simulink model "TSR_Scenario_001_cs"  (R2014b)
settings: Solver=ode5  SolverMode=SingleTasking  StartTime=0.0  StopTime=inf  FixedStep=1/100  RelTol=1e-3
PreLoadFcn:
  | mbxruntime.callbacks.PreLoadFcn(bdroot);
  | check_NUTS_defined;
  | 
  | assignin('base',['model_closed_' bdroot],false);
  | 
  | addpath('../includes_TSR/includes_TSR');
  | 
  | switch version('-release')
  | case {'2010a', '2010b', '2011a'}
  | addpath('../includes_TSR/ML2010b');
  | otherwise
  | addpath('../includes_TSR/ML2011b');
  | end
PostLoadFcn:
  | mbxruntime.callbacks.PostLoadFcn(bdroot);
InitFcn:
  | mbxruntime.callbacks.InitFcn(bdroot);
StartFcn:
  | mbxruntime.callbacks.StartFcn(bdroot);
StopFcn:
  | mbxruntime.callbacks.StopFcn(bdroot);
model workspace: external: MAT-File .\TSR_Scenario_001_cs_hws.mat (data not in the file)
undefined symbols (not defined in the file or in its folder): InitImageOutputDir, mbxruntime, OrientationPitch, OrientationRoll, PositionX, PositionY, PositionZ, tabledata, warningInitialVelocity, x0
undefined symbols (not defined in the file): SteeringColumn, SteeringWheel, TSR_Scenario_001_cs_0469e6db089af631, TSR_Scenario_001_cs_0511100212e7bc8e, TSR_Scenario_001_cs_0e7e9ae969427aac, TSR_Scenario_001_cs_1093386e49c2fe1f, TSR_Scenario_001_cs_112063adae8cf595, TSR_Scenario_001_cs_20f00d93cd5331c2, TSR_Scenario_001_cs_23e3512474fbfadc, TSR_Scenario_001_cs_366523e1554c6bf4, TSR_Scenario_001_cs_37bce4982c67337a, TSR_Scenario_001_cs_44e6164a5df50f45, TSR_Scenario_001_cs_4963ce12e7ff3247, TSR_Scenario_001_cs_4b3e01fa729ce73a, TSR_Scenario_001_cs_519c34727ce9f069, TSR_Scenario_001_cs_5b66ab60038399a1, TSR_Scenario_001_cs_5baa165dfa1afdcb, TSR_Scenario_001_cs_5f993ce39fa6372c, TSR_Scenario_001_cs_613fdf28e3ff7437, TSR_Scenario_001_cs_67b1406af835d622, TSR_Scenario_001_cs_6ad990c290286b94, TSR_Scenario_001_cs_6c412b69295984e1, TSR_Scenario_001_cs_6d4c0c06b1585ef3, TSR_Scenario_001_cs_6dd019d071bf1235, TSR_Scenario_001_cs_6e9f5883f1a78533, TSR_Scenario_001_cs_80f7223d9ac35404, TSR_Scenario_001_cs_8562b82d3c89ae57, TSR_Scenario_001_cs_8a3a0181ab0babfe, TSR_Scenario_001_cs_8c997348ce80deaf, TSR_Scenario_001_cs_925bd6a073d9fe25, TSR_Scenario_001_cs_961436216add6114, TSR_Scenario_001_cs_991a7959256b2c84, TSR_Scenario_001_cs_9a95ce2c2e753616, TSR_Scenario_001_cs_a98aa9562e8552a9, TSR_Scenario_001_cs_ab44ae81dbfb58cd, TSR_Scenario_001_cs_Actros_2541_2_Path_pathUniqueID, TSR_Scenario_001_cs_ae74836ade6bff5a, TSR_Scenario_001_cs_Audi_A8_1_Dynamics_Simple_initialPitch, TSR_Scenario_001_cs_Audi_A8_1_Dynamics_Simple_initialRoll, TSR_Scenario_001_cs_Audi_A8_1_Dynamics_Simple_initialX, TSR_Scenario_001_cs_Audi_A8_1_Dynamics_Simple_initialY, TSR_Scenario_001_cs_Audi_A8_1_Dynamics_Simple_initialYaw, TSR_Scenario_001_cs_Audi_A8_1_Dynamics_Simple_initialZ, TSR_Scenario_001_cs_Audi_A8_2_Path_pathUniqueID, TSR_Scenario_001_cs_Audi_A8_2_SpeedProfile_speedProfileUniqueID, TSR_Scenario_001_cs_b2eca4eb2fce349a, TSR_Scenario_001_cs_b7bac209c1f2549f, TSR_Scenario_001_cs_bf3dccb66d3255a4, TSR_Scenario_001_cs_bf4c1a5315e3f716, TSR_Scenario_001_cs_BMW_Z3_1_Path_pathUniqueID, TSR_Scenario_001_cs_BMW_Z3_1_SpeedProfile_speedProfileUniqueID, TSR_Scenario_001_cs_BMW_Z3_2_Path_pathUniqueID, TSR_Scenario_001_cs_BMW_Z3_2_SpeedProfile_speedProfileUniqueID, TSR_Scenario_001_cs_c4c8fc4bdece03a9, TSR_Scenario_001_cs_c964c86aa54ad92e, TSR_Scenario_001_cs_cb64d1ef85329755, TSR_Scenario_001_cs_Citroen_C3_1_Path_pathUniqueID, TSR_Scenario_001_cs_Citroen_C3_2_Path_pathUniqueID, TSR_Scenario_001_cs_Citroen_C3_3_Path_pathUniqueID, TSR_Scenario_001_cs_Citroen_C3_4_Path_pathUniqueID ... (+25)
libraries: simulink x21, PreScanSimulinkLibrary x17, simulink_extras x13
(part 14 of 30)

== system TSR_Scenario_001_cs/VISUMatrixSignLights_HighwayOverhang_2/Actuator ==
  VISUMatrixSignLights_HighwayOverhang_2 : Inport  Tag=inport/VisuMatrixSignLights  SampleTime=1/100  BusOutputAsStruct=on
  DemuxVisuLights : Demux  Outputs=16
  LimiterVisuLights : Saturate  UpperLimit=1  LowerLimit=0
  visu_MatrixSign_5_Light_1 : S-Function  FunctionName=sfun_MaterialColorSelector  Parameters=mbxruntime.parameters.convert(UniqueID), mbxruntime.parameters.convert(ColorsObjectQuery), mbxruntime.parameters.convert(Colors),tabledata, TimeStep  EnableBusSupport=off  mask(PreScan Sink Block: VisuMatrixSignLights){UniqueID=1877, ColorsObjectQuery=child:name=MatrixSign_5/child:name=HighwayOverhang_2.MatrixSign_5.OrangeLightUpperLeft, Colors=[32   25    5  255   64   48    5  255   64   54    5  255    0    0    0  255; 45   34    0  255   45   34    0  255   45   34    0  255  306  229    5  255], TimeStep=1/100}
      mask prompts: UniqueID "Parent Unique Identifier"; ColorsObjectQuery "Query for Color Object"; Colors "Matrix of colors"; TimeStep "Simulink time step"
      mask help:
      | The VisuMatrixSignLights block provides a way to switch the lights on the matrix sign board on or off
      |
      | For more information, please click Help.
      mask init:
      | [tabledata] = mbxruntime.parameters.table(UniqueID,ColorsObjectQuery,Colors);
      mask Help: eval('openHelp(732)')
      mask Display: image(imread('RearLight.png'))
  visu_MatrixSign_5_Light_2 : S-Function  FunctionName=sfun_MaterialColorSelector  Parameters=mbxruntime.parameters.convert(UniqueID), mbxruntime.parameters.convert(ColorsObjectQuery), mbxruntime.parameters.convert(Colors),tabledata, TimeStep  EnableBusSupport=off  mask(PreScan Sink Block: VisuMatrixSignLights){UniqueID=1877, ColorsObjectQuery=child:name=MatrixSign_5/child:name=HighwayOverhang_2.MatrixSign_5.OrangeLightUpperRight, Colors=[32   25    5  255   64   48    5  255   64   54    5  255    0    0    0  255; 45   34    0  255   45   34    0  255   45   34    0  255  306  229    5  255], TimeStep=1/100}
      mask prompts: UniqueID "Parent Unique Identifier"; ColorsObjectQuery "Query for Color Object"; Colors "Matrix of colors"; TimeStep "Simulink time step"
      mask help:
      | The VisuMatrixSignLights block provides a way to switch the lights on the matrix sign board on or off
      |
      | For more information, please click Help.
      mask init:
      | [tabledata] = mbxruntime.parameters.table(UniqueID,ColorsObjectQuery,Colors);
      mask Help: eval('openHelp(732)')
      mask Display: image(imread('RearLight.png'))
  visu_MatrixSign_5_Light_3 : S-Function  FunctionName=sfun_MaterialColorSelector  Parameters=mbxruntime.parameters.convert(UniqueID), mbxruntime.parameters.convert(ColorsObjectQuery), mbxruntime.parameters.convert(Colors),tabledata, TimeStep  EnableBusSupport=off  mask(PreScan Sink Block: VisuMatrixSignLights){UniqueID=1877, ColorsObjectQuery=child:name=MatrixSign_5/child:name=HighwayOverhang_2.MatrixSign_5.OrangeLightLowerLeft, Colors=[32   25    5  255   64   48    5  255   64   54    5  255    0    0    0  255; 45   34    0  255   45   34    0  255   45   34    0  255  306  229    5  255], TimeStep=1/100}
      mask prompts: UniqueID "Parent Unique Identifier"; ColorsObjectQuery "Query for Color Object"; Colors "Matrix of colors"; TimeStep "Simulink time step"
      mask help:
      | The VisuMatrixSignLights block provides a way to switch the lights on the matrix sign board on or off
      |
      | For more information, please click Help.
      mask init:
      | [tabledata] = mbxruntime.parameters.table(UniqueID,ColorsObjectQuery,Colors);
      mask Help: eval('openHelp(732)')
      mask Display: image(imread('RearLight.png'))
  visu_MatrixSign_5_Light_4 : S-Function  FunctionName=sfun_MaterialColorSelector  Parameters=mbxruntime.parameters.convert(UniqueID), mbxruntime.parameters.convert(ColorsObjectQuery), mbxruntime.parameters.convert(Colors),tabledata, TimeStep  EnableBusSupport=off  mask(PreScan Sink Block: VisuMatrixSignLights){UniqueID=1877, ColorsObjectQuery=child:name=MatrixSign_5/child:name=HighwayOverhang_2.MatrixSign_5.OrangeLightLowerRight, Colors=[32   25    5  255   64   48    5  255   64   54    5  255    0    0    0  255; 45   34    0  255   45   34    0  255   45   34    0  255  306  229    5  255], TimeStep=1/100}
      mask prompts: UniqueID "Parent Unique Identifier"; ColorsObjectQuery "Query for Color Object"; Colors "Matrix of colors"; TimeStep "Simulink time step"
      mask help:
      | The VisuMatrixSignLights block provides a way to switch the lights on the matrix sign board on or off
      |
      | For more information, please click Help.
      mask init:
      | [tabledata] = mbxruntime.parameters.table(UniqueID,ColorsObjectQuery,Colors);
      mask Help: eval('openHelp(732)')
      mask Display: image(imread('RearLight.png'))
  visu_MatrixSign_6_Light_1 : S-Function  FunctionName=sfun_MaterialColorSelector  Parameters=mbxruntime.parameters.convert(UniqueID), mbxruntime.parameters.convert(ColorsObjectQuery), mbxruntime.parameters.convert(Colors),tabledata, TimeStep  EnableBusSupport=off  mask(PreScan Sink Block: VisuMatrixSignLights){UniqueID=1877, ColorsObjectQuery=child:name=MatrixSign_6/child:name=HighwayOverhang_2.MatrixSign_6.OrangeLightUpperLeft, Colors=[32   25    5  255   64   48    5  255   64   54    5  255    0    0    0  255; 45   34    0  255   45   34    0  255   45   34    0  255  306  229    5  255], TimeStep=1/100}
      mask prompts: UniqueID "Parent Unique Identifier"; ColorsObjectQuery "Query for Color Object"; Colors "Matrix of colors"; TimeStep "Simulink time step"
      mask help:
      | The VisuMatrixSignLights block provides a way to switch the lights on the matrix sign board on or off
      |
      | For more information, please click Help.
      mask init:
      | [tabledata] = mbxruntime.parameters.table(UniqueID,ColorsObjectQuery,Colors);
      mask Help: eval('openHelp(732)')
      mask Display: image(imread('RearLight.png'))
  visu_MatrixSign_6_Light_2 : S-Function  FunctionName=sfun_MaterialColorSelector  Parameters=mbxruntime.parameters.convert(UniqueID), mbxruntime.parameters.convert(ColorsObjectQuery), mbxruntime.parameters.convert(Colors),tabledata, TimeStep  EnableBusSupport=off  mask(PreScan Sink Block: VisuMatrixSignLights){UniqueID=1877, ColorsObjectQuery=child:name=MatrixSign_6/child:name=HighwayOverhang_2.MatrixSign_6.OrangeLightUpperRight, Colors=[32   25    5  255   64   48    5  255   64   54    5  255    0    0    0  255; 45   34    0  255   45   34    0  255   45   34    0  255  306  229    5  255], TimeStep=1/100}
      mask prompts: UniqueID "Parent Unique Identifier"; ColorsObjectQuery "Query for Color Object"; Colors "Matrix of colors"; TimeStep "Simulink time step"
      mask help:
      | The VisuMatrixSignLights block provides a way to switch the lights on the matrix sign board on or off
      |
      | For more information, please click Help.
      mask init:
      | [tabledata] = mbxruntime.parameters.table(UniqueID,ColorsObjectQuery,Colors);
      mask Help: eval('openHelp(732)')
      mask Display: image(imread('RearLight.png'))
  visu_MatrixSign_6_Light_3 : S-Function  FunctionName=sfun_MaterialColorSelector  Parameters=mbxruntime.parameters.convert(UniqueID), mbxruntime.parameters.convert(ColorsObjectQuery), mbxruntime.parameters.convert(Colors),tabledata, TimeStep  EnableBusSupport=off  mask(PreScan Sink Block: VisuMatrixSignLights){UniqueID=1877, ColorsObjectQuery=child:name=MatrixSign_6/child:name=HighwayOverhang_2.MatrixSign_6.OrangeLightLowerLeft, Colors=[32   25    5  255   64   48    5  255   64   54    5  255    0    0    0  255; 45   34    0  255   45   34    0  255   45   34    0  255  306  229    5  255], TimeStep=1/100}
      mask prompts: UniqueID "Parent Unique Identifier"; ColorsObjectQuery "Query for Color Object"; Colors "Matrix of colors"; TimeStep "Simulink time step"
      mask help:
      | The VisuMatrixSignLights block provides a way to switch the lights on the matrix sign board on or off
      |
      | For more information, please click Help.
      mask init:
      | [tabledata] = mbxruntime.parameters.table(UniqueID,ColorsObjectQuery,Colors);
      mask Help: eval('openHelp(732)')
      mask Display: image(imread('RearLight.png'))
  visu_MatrixSign_6_Light_4 : S-Function  FunctionName=sfun_MaterialColorSelector  Parameters=mbxruntime.parameters.convert(UniqueID), mbxruntime.parameters.convert(ColorsObjectQuery), mbxruntime.parameters.convert(Colors),tabledata, TimeStep  EnableBusSupport=off  mask(PreScan Sink Block: VisuMatrixSignLights){UniqueID=1877, ColorsObjectQuery=child:name=MatrixSign_6/child:name=HighwayOverhang_2.MatrixSign_6.OrangeLightLowerRight, Colors=[32   25    5  255   64   48    5  255   64   54    5  255    0    0    0  255; 45   34    0  255   45   34    0  255   45   34    0  255  306  229    5  255], TimeStep=1/100}
      mask prompts: UniqueID "Parent Unique Identifier"; ColorsObjectQuery "Query for Color Object"; Colors "Matrix of colors"; TimeStep "Simulink time step"
      mask help:
      | The VisuMatrixSignLights block provides a way to switch the lights on the matrix sign board on or off
      |
      | For more information, please click Help.
      mask init:
      | [tabledata] = mbxruntime.parameters.table(UniqueID,ColorsObjectQuery,Colors);
      mask Help: eval('openHelp(732)')
      mask Display: image(imread('RearLight.png'))
  visu_MatrixSign_7_Light_1 : S-Function  FunctionName=sfun_MaterialColorSelector  Parameters=mbxruntime.parameters.convert(UniqueID), mbxruntime.parameters.convert(ColorsObjectQuery), mbxruntime.parameters.convert(Colors),tabledata, TimeStep  EnableBusSupport=off  mask(PreScan Sink Block: VisuMatrixSignLights){UniqueID=1877, ColorsObjectQuery=child:name=MatrixSign_7/child:name=HighwayOverhang_2.MatrixSign_7.OrangeLightUpperLeft, Colors=[32   25    5  255   64   48    5  255   64   54    5  255    0    0    0  255; 45   34    0  255   45   34    0  255   45   34    0  255  306  229    5  255], TimeStep=1/100}
      mask prompts: UniqueID "Parent Unique Identifier"; ColorsObjectQuery "Query for Color Object"; Colors "Matrix of colors"; TimeStep "Simulink time step"
      mask help:
      | The VisuMatrixSignLights block provides a way to switch the lights on the matrix sign board on or off
      |
      | For more information, please click Help.
      mask init:
      | [tabledata] = mbxruntime.parameters.table(UniqueID,ColorsObjectQuery,Colors);
      mask Help: eval('openHelp(732)')
      mask Display: image(imread('RearLight.png'))
  visu_MatrixSign_7_Light_2 : S-Function  FunctionName=sfun_MaterialColorSelector  Parameters=mbxruntime.parameters.convert(UniqueID), mbxruntime.parameters.convert(ColorsObjectQuery), mbxruntime.parameters.convert(Colors),tabledata, TimeStep  EnableBusSupport=off  mask(PreScan Sink Block: VisuMatrixSignLights){UniqueID=1877, ColorsObjectQuery=child:name=MatrixSign_7/child:name=HighwayOverhang_2.MatrixSign_7.OrangeLightUpperRight, Colors=[32   25    5  255   64   48    5  255   64   54    5  255    0    0    0  255; 45   34    0  255   45   34    0  255   45   34    0  255  306  229    5  255], TimeStep=1/100}
      mask prompts: UniqueID "Parent Unique Identifier"; ColorsObjectQuery "Query for Color Object"; Colors "Matrix of colors"; TimeStep "Simulink time step"
      mask help:
      | The VisuMatrixSignLights block provides a way to switch the lights on the matrix sign board on or off
      |
      | For more information, please click Help.
      mask init:
      | [tabledata] = mbxruntime.parameters.table(UniqueID,ColorsObjectQuery,Colors);
      mask Help: eval('openHelp(732)')
      mask Display: image(imread('RearLight.png'))
  visu_MatrixSign_7_Light_3 : S-Function  FunctionName=sfun_MaterialColorSelector  Parameters=mbxruntime.parameters.convert(UniqueID), mbxruntime.parameters.convert(ColorsObjectQuery), mbxruntime.parameters.convert(Colors),tabledata, TimeStep  EnableBusSupport=off  mask(PreScan Sink Block: VisuMatrixSignLights){UniqueID=1877, ColorsObjectQuery=child:name=MatrixSign_7/child:name=HighwayOverhang_2.MatrixSign_7.OrangeLightLowerLeft, Colors=[32   25    5  255   64   48    5  255   64   54    5  255    0    0    0  255; 45   34    0  255   45   34    0  255   45   34    0  255  306  229    5  255], TimeStep=1/100}
      mask prompts: UniqueID "Parent Unique Identifier"; ColorsObjectQuery "Query for Color Object"; Colors "Matrix of colors"; TimeStep "Simulink time step"
      mask help:
      | The VisuMatrixSignLights block provides a way to switch the lights on the matrix sign board on or off
      |
      | For more information, please click Help.
      mask init:
      | [tabledata] = mbxruntime.parameters.table(UniqueID,ColorsObjectQuery,Colors);
      mask Help: eval('openHelp(732)')
      mask Display: image(imread('RearLight.png'))
  visu_MatrixSign_7_Light_4 : S-Function  FunctionName=sfun_MaterialColorSelector  Parameters=mbxruntime.parameters.convert(UniqueID), mbxruntime.parameters.convert(ColorsObjectQuery), mbxruntime.parameters.convert(Colors),tabledata, TimeStep  EnableBusSupport=off  mask(PreScan Sink Block: VisuMatrixSignLights){UniqueID=1877, ColorsObjectQuery=child:name=MatrixSign_7/child:name=HighwayOverhang_2.MatrixSign_7.OrangeLightLowerRight, Colors=[32   25    5  255   64   48    5  255   64   54    5  255    0    0    0  255; 45   34    0  255   45   34    0  255   45   34    0  255  306  229    5  255], TimeStep=1/100}
      mask prompts: UniqueID "Parent Unique Identifier"; ColorsObjectQuery "Query for Color Object"; Colors "Matrix of colors"; TimeStep "Simulink time step"
      mask help:
      | The VisuMatrixSignLights block provides a way to switch the lights on the matrix sign board on or off
      |
      | For more information, please click Help.
      mask init:
      | [tabledata] = mbxruntime.parameters.table(UniqueID,ColorsObjectQuery,Colors);
      mask Help: eval('openHelp(732)')
      mask Display: image(imread('RearLight.png'))
  visu_MatrixSign_8_Light_1 : S-Function  FunctionName=sfun_MaterialColorSelector  Parameters=mbxruntime.parameters.convert(UniqueID), mbxruntime.parameters.convert(ColorsObjectQuery), mbxruntime.parameters.convert(Colors),tabledata, TimeStep  EnableBusSupport=off  mask(PreScan Sink Block: VisuMatrixSignLights){UniqueID=1877, ColorsObjectQuery=child:name=MatrixSign_8/child:name=HighwayOverhang_2.MatrixSign_8.OrangeLightUpperLeft, Colors=[32   25    5  255   64   48    5  255   64   54    5  255    0    0    0  255; 45   34    0  255   45   34    0  255   45   34    0  255  306  229    5  255], TimeStep=1/100}
      mask prompts: UniqueID "Parent Unique Identifier"; ColorsObjectQuery "Query for Color Object"; Colors "Matrix of colors"; TimeStep "Simulink time step"
      mask help:
      | The VisuMatrixSignLights block provides a way to switch the lights on the matrix sign board on or off
      |
      | For more information, please click Help.
      mask init:
      | [tabledata] = mbxruntime.parameters.table(UniqueID,ColorsObjectQuery,Colors);
      mask Help: eval('openHelp(732)')
      mask Display: image(imread('RearLight.png'))
  visu_MatrixSign_8_Light_2 : S-Function  FunctionName=sfun_MaterialColorSelector  Parameters=mbxruntime.parameters.convert(UniqueID), mbxruntime.parameters.convert(ColorsObjectQuery), mbxruntime.parameters.convert(Colors),tabledata, TimeStep  EnableBusSupport=off  mask(PreScan Sink Block: VisuMatrixSignLights){UniqueID=1877, ColorsObjectQuery=child:name=MatrixSign_8/child:name=HighwayOverhang_2.MatrixSign_8.OrangeLightUpperRight, Colors=[32   25    5  255   64   48    5  255   64   54    5  255    0    0    0  255; 45   34    0  255   45   34    0  255   45   34    0  255  306  229    5  255], TimeStep=1/100}
      mask prompts: UniqueID "Parent Unique Identifier"; ColorsObjectQuery "Query for Color Object"; Colors "Matrix of colors"; TimeStep "Simulink time step"
      mask help:
      | The VisuMatrixSignLights block provides a way to switch the lights on the matrix sign board on or off
      |
      | For more information, please click Help.
      mask init:
      | [tabledata] = mbxruntime.parameters.table(UniqueID,ColorsObjectQuery,Colors);
      mask Help: eval('openHelp(732)')
      mask Display: image(imread('RearLight.png'))
  visu_MatrixSign_8_Light_3 : S-Function  FunctionName=sfun_MaterialColorSelector  Parameters=mbxruntime.parameters.convert(UniqueID), mbxruntime.parameters.convert(ColorsObjectQuery), mbxruntime.parameters.convert(Colors),tabledata, TimeStep  EnableBusSupport=off  mask(PreScan Sink Block: VisuMatrixSignLights){UniqueID=1877, ColorsObjectQuery=child:name=MatrixSign_8/child:name=HighwayOverhang_2.MatrixSign_8.OrangeLightLowerLeft, Colors=[32   25    5  255   64   48    5  255   64   54    5  255    0    0    0  255; 45   34    0  255   45   34    0  255   45   34    0  255  306  229    5  255], TimeStep=1/100}
      mask prompts: UniqueID "Parent Unique Identifier"; ColorsObjectQuery "Query for Color Object"; Colors "Matrix of colors"; TimeStep "Simulink time step"
      mask help:
      | The VisuMatrixSignLights block provides a way to switch the lights on the matrix sign board on or off
      |
      | For more information, please click Help.
      mask init:
      | [tabledata] = mbxruntime.parameters.table(UniqueID,ColorsObjectQuery,Colors);
      mask Help: eval('openHelp(732)')
      mask Display: image(imread('RearLight.png'))
  visu_MatrixSign_8_Light_4 : S-Function  FunctionName=sfun_MaterialColorSelector  Parameters=mbxruntime.parameters.convert(UniqueID), mbxruntime.parameters.convert(ColorsObjectQuery), mbxruntime.parameters.convert(Colors),tabledata, TimeStep  EnableBusSupport=off  mask(PreScan Sink Block: VisuMatrixSignLights){UniqueID=1877, ColorsObjectQuery=child:name=MatrixSign_8/child:name=HighwayOverhang_2.MatrixSign_8.OrangeLightLowerRight, Colors=[32   25    5  255   64   48    5  255   64   54    5  255    0    0    0  255; 45   34    0  255   45   34    0  255   45   34    0  255  306  229    5  255], TimeStep=1/100}
      mask prompts: UniqueID "Parent Unique Identifier"; ColorsObjectQuery "Query for Color Object"; Colors "Matrix of colors"; TimeStep "Simulink time step"
      mask help:
      | The VisuMatrixSignLights block provides a way to switch the lights on the matrix sign board on or off
      |
      | For more information, please click Help.
      mask init:
      | [tabledata] = mbxruntime.parameters.table(UniqueID,ColorsObjectQuery,Colors);
      mask Help: eval('openHelp(732)')
      mask Display: image(imread('RearLight.png'))
  wires:
  VISUMatrixSignLights_HighwayOverhang_2/1 -> LimiterVisuLights/1
  LimiterVisuLights/1 -> DemuxVisuLights/1
  DemuxVisuLights/1 -> visu_MatrixSign_5_Light_1/1
  DemuxVisuLights/2 -> visu_MatrixSign_5_Light_2/1
  DemuxVisuLights/3 -> visu_MatrixSign_5_Light_3/1
  DemuxVisuLights/4 -> visu_MatrixSign_5_Light_4/1
  DemuxVisuLights/5 -> visu_MatrixSign_6_Light_1/1
  DemuxVisuLights/6 -> visu_MatrixSign_6_Light_2/1
  DemuxVisuLights/7 -> visu_MatrixSign_6_Light_3/1
  DemuxVisuLights/8 -> visu_MatrixSign_6_Light_4/1
  DemuxVisuLights/9 -> visu_MatrixSign_7_Light_1/1
  DemuxVisuLights/10 -> visu_MatrixSign_7_Light_2/1
  DemuxVisuLights/11 -> visu_MatrixSign_7_Light_3/1
  DemuxVisuLights/12 -> visu_MatrixSign_7_Light_4/1
  DemuxVisuLights/13 -> visu_MatrixSign_8_Light_1/1
  DemuxVisuLights/14 -> visu_MatrixSign_8_Light_2/1
  DemuxVisuLights/15 -> visu_MatrixSign_8_Light_3/1
  DemuxVisuLights/16 -> visu_MatrixSign_8_Light_4/1

== system TSR_Scenario_001_cs/VISUMatrixSignLights_HighwayOverhang_3/Actuator ==
  VISUMatrixSignLights_HighwayOverhang_3 : Inport  Tag=inport/VisuMatrixSignLights  SampleTime=1/100  BusOutputAsStruct=on
  DemuxVisuLights : Demux  Outputs=16
  LimiterVisuLights : Saturate  UpperLimit=1  LowerLimit=0
  visu_MatrixSign_10_Light_1 : S-Function  FunctionName=sfun_MaterialColorSelector  Parameters=mbxruntime.parameters.convert(UniqueID), mbxruntime.parameters.convert(ColorsObjectQuery), mbxruntime.parameters.convert(Colors),tabledata, TimeStep  EnableBusSupport=off  mask(PreScan Sink Block: VisuMatrixSignLights){UniqueID=1890, ColorsObjectQuery=child:name=MatrixSign_10/child:name=HighwayOverhang_3.MatrixSign_10.OrangeLightUpperLeft, Colors=[32   25    5  255   64   48    5  255   64   54    5  255    0    0    0  255; 45   34    0  255   45   34    0  255   45   34    0  255  306  229    5  255], TimeStep=1/100}
      mask prompts: UniqueID "Parent Unique Identifier"; ColorsObjectQuery "Query for Color Object"; Colors "Matrix of colors"; TimeStep "Simulink time step"
      mask help:
      | The VisuMatrixSignLights block provides a way to switch the lights on the matrix sign board on or off
      |
      | For more information, please click Help.
      mask init:
      | [tabledata] = mbxruntime.parameters.table(UniqueID,ColorsObjectQuery,Colors);
      mask Help: eval('openHelp(732)')
      mask Display: image(imread('RearLight.png'))
  visu_MatrixSign_10_Light_2 : S-Function  FunctionName=sfun_MaterialColorSelector  Parameters=mbxruntime.parameters.convert(UniqueID), mbxruntime.parameters.convert(ColorsObjectQuery), mbxruntime.parameters.convert(Colors),tabledata, TimeStep  EnableBusSupport=off  mask(PreScan Sink Block: VisuMatrixSignLights){UniqueID=1890, ColorsObjectQuery=child:name=MatrixSign_10/child:name=HighwayOverhang_3.MatrixSign_10.OrangeLightUpperRight, Colors=[32   25    5  255   64   48    5  255   64   54    5  255    0    0    0  255; 45   34    0  255   45   34    0  255   45   34    0  255  306  229    5  255], TimeStep=1/100}
      mask prompts: UniqueID "Parent Unique Identifier"; ColorsObjectQuery "Query for Color Object"; Colors "Matrix of colors"; TimeStep "Simulink time step"
      mask help:
      | The VisuMatrixSignLights block provides a way to switch the lights on the matrix sign board on or off
      |
      | For more information, please click Help.
      mask init:
      | [tabledata] = mbxruntime.parameters.table(UniqueID,ColorsObjectQuery,Colors);
      mask Help: eval('openHelp(732)')
      mask Display: image(imread('RearLight.png'))
  visu_MatrixSign_10_Light_3 : S-Function  FunctionName=sfun_MaterialColorSelector  Parameters=mbxruntime.parameters.convert(UniqueID), mbxruntime.parameters.convert(ColorsObjectQuery), mbxruntime.parameters.convert(Colors),tabledata, TimeStep  EnableBusSupport=off  mask(PreScan Sink Block: VisuMatrixSignLights){UniqueID=1890, ColorsObjectQuery=child:name=MatrixSign_10/child:name=HighwayOverhang_3.MatrixSign_10.OrangeLightLowerLeft, Colors=[32   25    5  255   64   48    5  255   64   54    5  255    0    0    0  255; 45   34    0  255   45   34    0  255   45   34    0  255  306  229    5  255], TimeStep=1/100}
      mask prompts: UniqueID "Parent Unique Identifier"; ColorsObjectQuery "Query for Color Object"; Colors "Matrix of colors"; TimeStep "Simulink time step"
      mask help:
      | The VisuMatrixSignLights block provides a way to switch the lights on the matrix sign board on or off
      |
      | For more information, please click Help.
      mask init:
      | [tabledata] = mbxruntime.parameters.table(UniqueID,ColorsObjectQuery,Colors);
      mask Help: eval('openHelp(732)')
      mask Display: image(imread('RearLight.png'))
  visu_MatrixSign_10_Light_4 : S-Function  FunctionName=sfun_MaterialColorSelector  Parameters=mbxruntime.parameters.convert(UniqueID), mbxruntime.parameters.convert(ColorsObjectQuery), mbxruntime.parameters.convert(Colors),tabledata, TimeStep  EnableBusSupport=off  mask(PreScan Sink Block: VisuMatrixSignLights){UniqueID=1890, ColorsObjectQuery=child:name=MatrixSign_10/child:name=HighwayOverhang_3.MatrixSign_10.OrangeLightLowerRight, Colors=[32   25    5  255   64   48    5  255   64   54    5  255    0    0    0  255; 45   34    0  255   45   34    0  255   45   34    0  255  306  229    5  255], TimeStep=1/100}
      mask prompts: UniqueID "Parent Unique Identifier"; ColorsObjectQuery "Query for Color Object"; Colors "Matrix of colors"; TimeStep "Simulink time step"
      mask help:
      | The VisuMatrixSignLights block provides a way to switch the lights on the matrix sign board on or off
      |
      | For more information, please click Help.
      mask init:
      | [tabledata] = mbxruntime.parameters.table(UniqueID,ColorsObjectQuery,Colors);
      mask Help: eval('openHelp(732)')
      mask Display: image(imread('RearLight.png'))
  visu_MatrixSign_11_Light_1 : S-Function  FunctionName=sfun_MaterialColorSelector  Parameters=mbxruntime.parameters.convert(UniqueID), mbxruntime.parameters.convert(ColorsObjectQuery), mbxruntime.parameters.convert(Colors),tabledata, TimeStep  EnableBusSupport=off  mask(PreScan Sink Block: VisuMatrixSignLights){UniqueID=1890, ColorsObjectQuery=child:name=MatrixSign_11/child:name=HighwayOverhang_3.MatrixSign_11.OrangeLightUpperLeft, Colors=[32   25    5  255   64   48    5  255   64   54    5  255    0    0    0  255; 45   34    0  255   45   34    0  255   45   34    0  255  306  229    5  255], TimeStep=1/100}
      mask prompts: UniqueID "Parent Unique Identifier"; ColorsObjectQuery "Query for Color Object"; Colors "Matrix of colors"; TimeStep "Simulink time step"
      mask help:
      | The VisuMatrixSignLights block provides a way to switch the lights on the matrix sign board on or off
      |
      | For more information, please click Help.
      mask init:
      | [tabledata] = mbxruntime.parameters.table(UniqueID,ColorsObjectQuery,Colors);
      mask Help: eval('openHelp(732)')
      mask Display: image(imread('RearLight.png'))
  visu_MatrixSign_11_Light_2 : S-Function  FunctionName=sfun_MaterialColorSelector  Parameters=mbxruntime.parameters.convert(UniqueID), mbxruntime.parameters.convert(ColorsObjectQuery), mbxruntime.parameters.convert(Colors),tabledata, TimeStep  EnableBusSupport=off  mask(PreScan Sink Block: VisuMatrixSignLights){UniqueID=1890, ColorsObjectQuery=child:name=MatrixSign_11/child:name=HighwayOverhang_3.MatrixSign_11.OrangeLightUpperRight, Colors=[32   25    5  255   64   48    5  255   64   54    5  255    0    0    0  255; 45   34    0  255   45   34    0  255   45   34    0  255  306  229    5  255], TimeStep=1/100}
      mask prompts: UniqueID "Parent Unique Identifier"; ColorsObjectQuery "Query for Color Object"; Colors "Matrix of colors"; TimeStep "Simulink time step"
      mask help:
      | The VisuMatrixSignLights block provides a way to switch the lights on the matrix sign board on or off
      |
      | For more information, please click Help.
      mask init:
      | [tabledata] = mbxruntime.parameters.table(UniqueID,ColorsObjectQuery,Colors);
      mask Help: eval('openHelp(732)')
      mask Display: image(imread('RearLight.png'))
  visu_MatrixSign_11_Light_3 : S-Function  FunctionName=sfun_MaterialColorSelector  Parameters=mbxruntime.parameters.convert(UniqueID), mbxruntime.parameters.convert(ColorsObjectQuery), mbxruntime.parameters.convert(Colors),tabledata, TimeStep  EnableBusSupport=off  mask(PreScan Sink Block: VisuMatrixSignLights){UniqueID=1890, ColorsObjectQuery=child:name=MatrixSign_11/child:name=HighwayOverhang_3.MatrixSign_11.OrangeLightLowerLeft, Colors=[32   25    5  255   64   48    5  255   64   54    5  255    0    0    0  255; 45   34    0  255   45   34    0  255   45   34    0  255  306  229    5  255], TimeStep=1/100}
      mask prompts: UniqueID "Parent Unique Identifier"; ColorsObjectQuery "Query for Color Object"; Colors "Matrix of colors"; TimeStep "Simulink time step"
      mask help:
      | The VisuMatrixSignLights block provides a way to switch the lights on the matrix sign board on or off
      |
      | For more information, please click Help.
      mask init:
      | [tabledata] = mbxruntime.parameters.table(UniqueID,ColorsObjectQuery,Colors);
      mask Help: eval('openHelp(732)')
      mask Display: image(imread('RearLight.png'))
  visu_MatrixSign_11_Light_4 : S-Function  FunctionName=sfun_MaterialColorSelector  Parameters=mbxruntime.parameters.convert(UniqueID), mbxruntime.parameters.convert(ColorsObjectQuery), mbxruntime.parameters.convert(Colors),tabledata, TimeStep  EnableBusSupport=off  mask(PreScan Sink Block: VisuMatrixSignLights){UniqueID=1890, ColorsObjectQuery=child:name=MatrixSign_11/child:name=HighwayOverhang_3.MatrixSign_11.OrangeLightLowerRight, Colors=[32   25    5  255   64   48    5  255   64   54    5  255    0    0    0  255; 45   34    0  255   45   34    0  255   45   34    0  255  306  229    5  255], TimeStep=1/100}
      mask prompts: UniqueID "Parent Unique Identifier"; ColorsObjectQuery "Query for Color Object"; Colors "Matrix of colors"; TimeStep "Simulink time step"
      mask help:
      | The VisuMatrixSignLights block provides a way to switch the lights on the matrix sign board on or off
      |
      | For more information, please click Help.
      mask init:
      | [tabledata] = mbxruntime.parameters.table(UniqueID,ColorsObjectQuery,Colors);
      mask Help: eval('openHelp(732)')
      mask Display: image(imread('RearLight.png'))
  visu_MatrixSign_12_Light_1 : S-Function  FunctionName=sfun_MaterialColorSelector  Parameters=mbxruntime.parameters.convert(UniqueID), mbxruntime.parameters.convert(ColorsObjectQuery), mbxruntime.parameters.convert(Colors),tabledata, TimeStep  EnableBusSupport=off  mask(PreScan Sink Block: VisuMatrixSignLights){UniqueID=1890, ColorsObjectQuery=child:name=MatrixSign_12/child:name=HighwayOverhang_3.MatrixSign_12.OrangeLightUpperLeft, Colors=[32   25    5  255   64   48    5  255   64   54    5  255    0    0    0  255; 45   34    0  255   45   34    0  255   45   34    0  255  306  229    5  255], TimeStep=1/100}
      mask prompts: UniqueID "Parent Unique Identifier"; ColorsObjectQuery "Query for Color Object"; Colors "Matrix of colors"; TimeStep "Simulink time step"
      mask help:
      | The VisuMatrixSignLights block provides a way to switch the lights on the matrix sign board on or off
      |
      | For more information, please click Help.
      mask init:
      | [tabledata] = mbxruntime.parameters.table(UniqueID,ColorsObjectQuery,Colors);
      mask Help: eval('openHelp(732)')
      mask Display: image(imread('RearLight.png'))
  visu_MatrixSign_12_Light_2 : S-Function  FunctionName=sfun_MaterialColorSelector  Parameters=mbxruntime.parameters.convert(UniqueID), mbxruntime.parameters.convert(ColorsObjectQuery), mbxruntime.parameters.convert(Colors),tabledata, TimeStep  EnableBusSupport=off  mask(PreScan Sink Block: VisuMatrixSignLights){UniqueID=1890, ColorsObjectQuery=child:name=MatrixSign_12/child:name=HighwayOverhang_3.MatrixSign_12.OrangeLightUpperRight, Colors=[32   25    5  255   64   48    5  255   64   54    5  255    0    0    0  255; 45   34    0  255   45   34    0  255   45   34    0  255  306  229    5  255], TimeStep=1/100}
      mask prompts: UniqueID "Parent Unique Identifier"; ColorsObjectQuery "Query for Color Object"; Colors "Matrix of colors"; TimeStep "Simulink time step"
      mask help:
      | The VisuMatrixSignLights block provides a way to switch the lights on the matrix sign board on or off
      |
      | For more information, please click Help.
      mask init:
      | [tabledata] = mbxruntime.parameters.table(UniqueID,ColorsObjectQuery,Colors);
      mask Help: eval('openHelp(732)')
      mask Display: image(imread('RearLight.png'))
  visu_MatrixSign_12_Light_3 : S-Function  FunctionName=sfun_MaterialColorSelector  Parameters=mbxruntime.parameters.convert(UniqueID), mbxruntime.parameters.convert(ColorsObjectQuery), mbxruntime.parameters.convert(Colors),tabledata, TimeStep  EnableBusSupport=off  mask(PreScan Sink Block: VisuMatrixSignLights){UniqueID=1890, ColorsObjectQuery=child:name=MatrixSign_12/child:name=HighwayOverhang_3.MatrixSign_12.OrangeLightLowerLeft, Colors=[32   25    5  255   64   48    5  255   64   54    5  255    0    0    0  255; 45   34    0  255   45   34    0  255   45   34    0  255  306  229    5  255], TimeStep=1/100}
      mask prompts: UniqueID "Parent Unique Identifier"; ColorsObjectQuery "Query for Color Object"; Colors "Matrix of colors"; TimeStep "Simulink time step"
      mask help:
      | The VisuMatrixSignLights block provides a way to switch the lights on the matrix sign board on or off
      |
      | For more information, please click Help.
      mask init:
      | [tabledata] = mbxruntime.parameters.table(UniqueID,ColorsObjectQuery,Colors);
      mask Help: eval('openHelp(732)')
      mask Display: image(imread('RearLight.png'))
  visu_MatrixSign_12_Light_4 : S-Function  FunctionName=sfun_MaterialColorSelector  Parameters=mbxruntime.parameters.convert(UniqueID), mbxruntime.parameters.convert(ColorsObjectQuery), mbxruntime.parameters.convert(Colors),tabledata, TimeStep  EnableBusSupport=off  mask(PreScan Sink Block: VisuMatrixSignLights){UniqueID=1890, ColorsObjectQuery=child:name=MatrixSign_12/child:name=HighwayOverhang_3.MatrixSign_12.OrangeLightLowerRight, Colors=[32   25    5  255   64   48    5  255   64   54    5  255    0    0    0  255; 45   34    0  255   45   34    0  255   45   34    0  255  306  229    5  255], TimeStep=1/100}
      mask prompts: UniqueID "Parent Unique Identifier"; ColorsObjectQuery "Query for Color Object"; Colors "Matrix of colors"; TimeStep "Simulink time step"
      mask help:
      | The VisuMatrixSignLights block provides a way to switch the lights on the matrix sign board on or off
      |
      | For more information, please click Help.
      mask init:
      | [tabledata] = mbxruntime.parameters.table(UniqueID,ColorsObjectQuery,Colors);
      mask Help: eval('openHelp(732)')
      mask Display: image(imread('RearLight.png'))
  visu_MatrixSign_9_Light_1 : S-Function  FunctionName=sfun_MaterialColorSelector  Parameters=mbxruntime.parameters.convert(UniqueID), mbxruntime.parameters.convert(ColorsObjectQuery), mbxruntime.parameters.convert(Colors),tabledata, TimeStep  EnableBusSupport=off  mask(PreScan Sink Block: VisuMatrixSignLights){UniqueID=1890, ColorsObjectQuery=child:name=MatrixSign_9/child:name=HighwayOverhang_3.MatrixSign_9.OrangeLightUpperLeft, Colors=[32   25    5  255   64   48    5  255   64   54    5  255    0    0    0  255; 45   34    0  255   45   34    0  255   45   34    0  255  306  229    5  255], TimeStep=1/100}
      mask prompts: UniqueID "Parent Unique Identifier"; ColorsObjectQuery "Query for Color Object"; Colors "Matrix of colors"; TimeStep "Simulink time step"
      mask help:
      | The VisuMatrixSignLights block provides a way to switch the lights on the matrix sign board on or off
      |
      | For more information, please click Help.
      mask init:
      | [tabledata] = mbxruntime.parameters.table(UniqueID,ColorsObjectQuery,Colors);
      mask Help: eval('openHelp(732)')
      mask Display: image(imread('RearLight.png'))
  visu_MatrixSign_9_Light_2 : S-Function  FunctionName=sfun_MaterialColorSelector  Parameters=mbxruntime.parameters.convert(UniqueID), mbxruntime.parameters.convert(ColorsObjectQuery), mbxruntime.parameters.convert(Colors),tabledata, TimeStep  EnableBusSupport=off  mask(PreScan Sink Block: VisuMatrixSignLights){UniqueID=1890, ColorsObjectQuery=child:name=MatrixSign_9/child:name=HighwayOverhang_3.MatrixSign_9.OrangeLightUpperRight, Colors=[32   25    5  255   64   48    5  255   64   54    5  255    0    0    0  255; 45   34    0  255   45   34    0  255   45   34    0  255  306  229    5  255], TimeStep=1/100}
      mask prompts: UniqueID "Parent Unique Identifier"; ColorsObjectQuery "Query for Color Object"; Colors "Matrix of colors"; TimeStep "Simulink time step"
      mask help:
      | The VisuMatrixSignLights block provides a way to switch the lights on the matrix sign board on or off
      |
      | For more information, please click Help.
      mask init:
      | [tabledata] = mbxruntime.parameters.table(UniqueID,ColorsObjectQuery,Colors);
      mask Help: eval('openHelp(732)')
      mask Display: image(imread('RearLight.png'))
  visu_MatrixSign_9_Light_3 : S-Function  FunctionName=sfun_MaterialColorSelector  Parameters=mbxruntime.parameters.convert(UniqueID), mbxruntime.parameters.convert(ColorsObjectQuery), mbxruntime.parameters.convert(Colors),tabledata, TimeStep  EnableBusSupport=off  mask(PreScan Sink Block: VisuMatrixSignLights){UniqueID=1890, ColorsObjectQuery=child:name=MatrixSign_9/child:name=HighwayOverhang_3.MatrixSign_9.OrangeLightLowerLeft, Colors=[32   25    5  255   64   48    5  255   64   54    5  255    0    0    0  255; 45   34    0  255   45   34    0  255   45   34    0  255  306  229    5  255], TimeStep=1/100}
      mask prompts: UniqueID "Parent Unique Identifier"; ColorsObjectQuery "Query for Color Object"; Colors "Matrix of colors"; TimeStep "Simulink time step"
      mask help:
      | The VisuMatrixSignLights block provides a way to switch the lights on the matrix sign board on or off
      |
      | For more information, please click Help.
      mask init:
      | [tabledata] = mbxruntime.parameters.table(UniqueID,ColorsObjectQuery,Colors);
      mask Help: eval('openHelp(732)')
      mask Display: image(imread('RearLight.png'))
  visu_MatrixSign_9_Light_4 : S-Function  FunctionName=sfun_MaterialColorSelector  Parameters=mbxruntime.parameters.convert(UniqueID), mbxruntime.parameters.convert(ColorsObjectQuery), mbxruntime.parameters.convert(Colors),tabledata, TimeStep  EnableBusSupport=off  mask(PreScan Sink Block: VisuMatrixSignLights){UniqueID=1890, ColorsObjectQuery=child:name=MatrixSign_9/child:name=HighwayOverhang_3.MatrixSign_9.OrangeLightLowerRight, Colors=[32   25    5  255   64   48    5  255   64   54    5  255    0    0    0  255; 45   34    0  255   45   34    0  255   45   34    0  255  306  229    5  255], TimeStep=1/100}
      mask prompts: UniqueID "Parent Unique Identifier"; ColorsObjectQuery "Query for Color Object"; Colors "Matrix of colors"; TimeStep "Simulink time step"
      mask help:
      | The VisuMatrixSignLights block provides a way to switch the lights on the matrix sign board on or off
      |
      | For more information, please click Help.
      mask init:
      | [tabledata] = mbxruntime.parameters.table(UniqueID,ColorsObjectQuery,Colors);
      mask Help: eval('openHelp(732)')
      mask Display: image(imread('RearLight.png'))
  wires:
  VISUMatrixSignLights_HighwayOverhang_3/1 -> LimiterVisuLights/1
  LimiterVisuLights/1 -> DemuxVisuLights/1
  DemuxVisuLights/1 -> visu_MatrixSign_9_Light_1/1
  DemuxVisuLights/2 -> visu_MatrixSign_9_Light_2/1
  DemuxVisuLights/3 -> visu_MatrixSign_9_Light_3/1
  DemuxVisuLights/4 -> visu_MatrixSign_9_Light_4/1
  DemuxVisuLights/5 -> visu_MatrixSign_10_Light_1/1
  DemuxVisuLights/6 -> visu_MatrixSign_10_Light_2/1
  DemuxVisuLights/7 -> visu_MatrixSign_10_Light_3/1
  DemuxVisuLights/8 -> visu_MatrixSign_10_Light_4/1
  DemuxVisuLights/9 -> visu_MatrixSign_11_Light_1/1
  DemuxVisuLights/10 -> visu_MatrixSign_11_Light_2/1
  DemuxVisuLights/11 -> visu_MatrixSign_11_Light_3/1
  DemuxVisuLights/12 -> visu_MatrixSign_11_Light_4/1
  DemuxVisuLights/13 -> visu_MatrixSign_12_Light_1/1
  DemuxVisuLights/14 -> visu_MatrixSign_12_Light_2/1
  DemuxVisuLights/15 -> visu_MatrixSign_12_Light_3/1
  DemuxVisuLights/16 -> visu_MatrixSign_12_Light_4/1
